simulink model "generic_uservehicle_truck"  (Simulink 10.3)
settings: Solver=ode45  StartTime=0.0  StopTime=inf  RelTol=1e-3  EnableMultiTasking=on
(part 4 of 4)

== system generic_uservehicle_truck/TruckMaker/Vehicle/IPG Vehicle/CarAndTrailer/Trailer/CreateBus Vhcl.Wheel.RL2 ==
  In1 : Inport
  Bus Creator3 : BusCreator  Inputs=14
  Demux3 : Demux  Outputs=14
      settings: DisplayOption=none
  Out1 : Outport  VectorParamsAs1DForOutWhenUnconnected=off
  wires:
  Demux3/14 -> Bus Creator3/14  "Vhcl Wheel RL2 Trq_WhlBearing"
  Demux3/13 -> Bus Creator3/13  "Vhcl Wheel RL2 Trq_T2W"
  Demux3/12 -> Bus Creator3/12  "Vhcl Wheel RL2 SideSlip"
  Demux3/11 -> Bus Creator3/11  "Vhcl Wheel RL2 LongSlip"
  Demux3/10 -> Bus Creator3/10  "Vhcl Wheel RL2 vBelt"
  Demux3/9 -> Bus Creator3/9  "Vhcl Wheel RL2 Fz"
  Demux3/8 -> Bus Creator3/8  "Vhcl Wheel RL2 Fy"
  Demux3/7 -> Bus Creator3/7  "Vhcl Wheel RL2 Fx"
  Demux3/6 -> Bus Creator3/6  "Vhcl Wheel RL2 r_zxy z"
  Demux3/5 -> Bus Creator3/5  "Vhcl Wheel RL2 r_zxy y"
  Demux3/4 -> Bus Creator3/4  "Vhcl Wheel RL2 r_zxy x"
  Demux3/3 -> Bus Creator3/3  "Vhcl Wheel RL2 t z"
  Demux3/2 -> Bus Creator3/2  "Vhcl Wheel RL2 t y"
  In1/1 -> Demux3/1
  Bus Creator3/1 -> Out1/1
  Demux3/1 -> Bus Creator3/1  "Vhcl Wheel RL2 t x"

== system generic_uservehicle_truck/TruckMaker/Vehicle/IPG Vehicle/CarAndTrailer/Trailer/CreateBus Vhcl.Wheel.RL3 ==
  In1 : Inport
  Bus Creator3 : BusCreator  Inputs=14
  Demux3 : Demux  Outputs=14
      settings: DisplayOption=none
  Out1 : Outport  VectorParamsAs1DForOutWhenUnconnected=off
  wires:
  Demux3/1 -> Bus Creator3/1  "Vhcl Wheel RL3 t x"
  Bus Creator3/1 -> Out1/1
  In1/1 -> Demux3/1
  Demux3/2 -> Bus Creator3/2  "Vhcl Wheel RL3 t y"
  Demux3/3 -> Bus Creator3/3  "Vhcl Wheel RL3 t z"
  Demux3/4 -> Bus Creator3/4  "Vhcl Wheel RL3 r_zxy x"
  Demux3/5 -> Bus Creator3/5  "Vhcl Wheel RL3 r_zxy y"
  Demux3/6 -> Bus Creator3/6  "Vhcl Wheel RL3 r_zxy z"
  Demux3/7 -> Bus Creator3/7  "Vhcl Wheel RL3 Fx"
  Demux3/8 -> Bus Creator3/8  "Vhcl Wheel RL3 Fy"
  Demux3/9 -> Bus Creator3/9  "Vhcl Wheel RL3 Fz"
  Demux3/10 -> Bus Creator3/10  "Vhcl Wheel RL3 vBelt"
  Demux3/11 -> Bus Creator3/11  "Vhcl Wheel RL3 LongSlip"
  Demux3/12 -> Bus Creator3/12  "Vhcl Wheel RL3 SideSlip"
  Demux3/13 -> Bus Creator3/13  "Vhcl Wheel RL3 Trq_T2W"
  Demux3/14 -> Bus Creator3/14  "Vhcl Wheel RL3 Trq_WhlBearing"

== system generic_uservehicle_truck/TruckMaker/Vehicle/IPG Vehicle/CarAndTrailer/Trailer/CreateBus Vhcl.Wheel.RL4 ==
  In1 : Inport
  Bus Creator3 : BusCreator  Inputs=14
  Demux3 : Demux  Outputs=14
      settings: DisplayOption=none
  Out1 : Outport  VectorParamsAs1DForOutWhenUnconnected=off
  wires:
  Demux3/14 -> Bus Creator3/14  "Vhcl Wheel RL4 Trq_WhlBearing"
  Demux3/13 -> Bus Creator3/13  "Vhcl Wheel RL4 Trq_T2W"
  Demux3/12 -> Bus Creator3/12  "Vhcl Wheel RL4 SideSlip"
  Demux3/11 -> Bus Creator3/11  "Vhcl Wheel RL4 LongSlip"
  Demux3/10 -> Bus Creator3/10  "Vhcl Wheel RL4 vBelt"
  Demux3/9 -> Bus Creator3/9  "Vhcl Wheel RL4 Fz"
  Demux3/8 -> Bus Creator3/8  "Vhcl Wheel RL4 Fy"
  Demux3/7 -> Bus Creator3/7  "Vhcl Wheel RL4 Fx"
  Demux3/6 -> Bus Creator3/6  "Vhcl Wheel RL4 r_zxy z"
  Demux3/5 -> Bus Creator3/5  "Vhcl Wheel RL4 r_zxy y"
  Demux3/4 -> Bus Creator3/4  "Vhcl Wheel RL4 r_zxy x"
  Demux3/3 -> Bus Creator3/3  "Vhcl Wheel RL4 t z"
  Demux3/2 -> Bus Creator3/2  "Vhcl Wheel RL4 t y"
  In1/1 -> Demux3/1
  Bus Creator3/1 -> Out1/1
  Demux3/1 -> Bus Creator3/1  "Vhcl Wheel RL4 t x"

== system generic_uservehicle_truck/TruckMaker/Vehicle/IPG Vehicle/CarAndTrailer/Trailer/CreateBus Vhcl.Wheel.RR ==
  In1 : Inport
  Bus Creator3 : BusCreator  Inputs=14
  Demux3 : Demux  Outputs=14
      settings: DisplayOption=none
  Out1 : Outport  VectorParamsAs1DForOutWhenUnconnected=off
  wires:
  Demux3/14 -> Bus Creator3/14  "Vhcl Wheel RR Trq_WhlBearing"
  Demux3/13 -> Bus Creator3/13  "Vhcl Wheel RR Trq_T2W"
  Demux3/12 -> Bus Creator3/12  "Vhcl Wheel RR SideSlip"
  Demux3/11 -> Bus Creator3/11  "Vhcl Wheel RR LongSlip"
  Demux3/10 -> Bus Creator3/10  "Vhcl Wheel RR vBelt"
  Demux3/9 -> Bus Creator3/9  "Vhcl Wheel RR Fz"
  Demux3/8 -> Bus Creator3/8  "Vhcl Wheel RR Fy"
  Demux3/7 -> Bus Creator3/7  "Vhcl Wheel RR Fx"
  Demux3/6 -> Bus Creator3/6  "Vhcl Wheel RR r_zxy z"
  Demux3/5 -> Bus Creator3/5  "Vhcl Wheel RR r_zxy y"
  Demux3/4 -> Bus Creator3/4  "Vhcl Wheel RR r_zxy x"
  Demux3/3 -> Bus Creator3/3  "Vhcl Wheel RR t z"
  Demux3/2 -> Bus Creator3/2  "Vhcl Wheel RR t y"
  In1/1 -> Demux3/1
  Bus Creator3/1 -> Out1/1
  Demux3/1 -> Bus Creator3/1  "Vhcl Wheel RR t x"

== system generic_uservehicle_truck/TruckMaker/Vehicle/IPG Vehicle/CarAndTrailer/Trailer/CreateBus Vhcl.Wheel.RR2 ==
  In1 : Inport
  Bus Creator3 : BusCreator  Inputs=14
  Demux3 : Demux  Outputs=14
      settings: DisplayOption=none
  Out1 : Outport  VectorParamsAs1DForOutWhenUnconnected=off
  wires:
  Demux3/14 -> Bus Creator3/14  "Vhcl Wheel RR2 Trq_WhlBearing"
  Demux3/13 -> Bus Creator3/13  "Vhcl Wheel RR2 Trq_T2W"
  Demux3/12 -> Bus Creator3/12  "Vhcl Wheel RR2 SideSlip"
  Demux3/11 -> Bus Creator3/11  "Vhcl Wheel RR2 LongSlip"
  Demux3/10 -> Bus Creator3/10  "Vhcl Wheel RR2 vBelt"
  Demux3/9 -> Bus Creator3/9  "Vhcl Wheel RR2 Fz"
  Demux3/8 -> Bus Creator3/8  "Vhcl Wheel RR2 Fy"
  Demux3/7 -> Bus Creator3/7  "Vhcl Wheel RR2 Fx"
  Demux3/6 -> Bus Creator3/6  "Vhcl Wheel RR2 r_zxy z"
  Demux3/5 -> Bus Creator3/5  "Vhcl Wheel RR2 r_zxy y"
  Demux3/4 -> Bus Creator3/4  "Vhcl Wheel RR2 r_zxy x"
  Demux3/3 -> Bus Creator3/3  "Vhcl Wheel RR2 t z"
  Demux3/2 -> Bus Creator3/2  "Vhcl Wheel RR2 t y"
  In1/1 -> Demux3/1
  Bus Creator3/1 -> Out1/1
  Demux3/1 -> Bus Creator3/1  "Vhcl Wheel RR2 t x"

== system generic_uservehicle_truck/TruckMaker/Vehicle/IPG Vehicle/CarAndTrailer/Trailer/CreateBus Vhcl.Wheel.RR3 ==
  In1 : Inport
  Bus Creator3 : BusCreator  Inputs=14
  Demux3 : Demux  Outputs=14
      settings: DisplayOption=none
  Out1 : Outport  VectorParamsAs1DForOutWhenUnconnected=off
  wires:
  Demux3/1 -> Bus Creator3/1  "Vhcl Wheel RR3 t x"
  Bus Creator3/1 -> Out1/1
  In1/1 -> Demux3/1
  Demux3/2 -> Bus Creator3/2  "Vhcl Wheel RR3 t y"
  Demux3/3 -> Bus Creator3/3  "Vhcl Wheel RR3 t z"
  Demux3/4 -> Bus Creator3/4  "Vhcl Wheel RR3 r_zxy x"
  Demux3/5 -> Bus Creator3/5  "Vhcl Wheel RR3 r_zxy y"
  Demux3/6 -> Bus Creator3/6  "Vhcl Wheel RR3 r_zxy z"
  Demux3/7 -> Bus Creator3/7  "Vhcl Wheel RR3 Fx"
  Demux3/8 -> Bus Creator3/8  "Vhcl Wheel RR3 Fy"
  Demux3/9 -> Bus Creator3/9  "Vhcl Wheel RR3 Fz"
  Demux3/10 -> Bus Creator3/10  "Vhcl Wheel RR3 vBelt"
  Demux3/11 -> Bus Creator3/11  "Vhcl Wheel RR3 LongSlip"
  Demux3/12 -> Bus Creator3/12  "Vhcl Wheel RR3 SideSlip"
  Demux3/13 -> Bus Creator3/13  "Vhcl Wheel RR3 Trq_T2W"
  Demux3/14 -> Bus Creator3/14  "Vhcl Wheel RR3 Trq_WhlBearing"

== system generic_uservehicle_truck/TruckMaker/Vehicle/IPG Vehicle/CarAndTrailer/Trailer/CreateBus Vhcl.Wheel.RR4 ==
  In1 : Inport
  Bus Creator3 : BusCreator  Inputs=14
  Demux3 : Demux  Outputs=14
      settings: DisplayOption=none
  Out1 : Outport  VectorParamsAs1DForOutWhenUnconnected=off
  wires:
  Demux3/14 -> Bus Creator3/14  "Vhcl Wheel RR4 Trq_WhlBearing"
  Demux3/13 -> Bus Creator3/13  "Vhcl Wheel RR4 Trq_T2W"
  Demux3/12 -> Bus Creator3/12  "Vhcl Wheel RR4 SideSlip"
  Demux3/11 -> Bus Creator3/11  "Vhcl Wheel RR4 LongSlip"
  Demux3/10 -> Bus Creator3/10  "Vhcl Wheel RR4 vBelt"
  Demux3/9 -> Bus Creator3/9  "Vhcl Wheel RR4 Fz"
  Demux3/8 -> Bus Creator3/8  "Vhcl Wheel RR4 Fy"
  Demux3/7 -> Bus Creator3/7  "Vhcl Wheel RR4 Fx"
  Demux3/6 -> Bus Creator3/6  "Vhcl Wheel RR4 r_zxy z"
  Demux3/5 -> Bus Creator3/5  "Vhcl Wheel RR4 r_zxy y"
  Demux3/4 -> Bus Creator3/4  "Vhcl Wheel RR4 r_zxy x"
  Demux3/3 -> Bus Creator3/3  "Vhcl Wheel RR4 t z"
  Demux3/2 -> Bus Creator3/2  "Vhcl Wheel RR4 t y"
  In1/1 -> Demux3/1
  Bus Creator3/1 -> Out1/1
  Demux3/1 -> Bus Creator3/1  "Vhcl Wheel RR4 t x"

== system generic_uservehicle_truck/TruckMaker/Vehicle/User Vehicle (CM4SL)/CarAndTrailer/CarAndTrailerUpd/CreateBus Brake.IF.In ==
  In : Inport
  BusCreator : BusCreator  Inputs=25
  Demux : Demux  Outputs=25
      settings: DisplayOption=none
  Out : Outport  VectorParamsAs1DForOutWhenUnconnected=off
  wires:
  Demux/25 -> BusCreator/25  "Brake IF Trq_Reg RR4"
  Demux/24 -> BusCreator/24  "Brake IF Trq_Reg RL4"
  Demux/23 -> BusCreator/23  "Brake IF Trq_Reg RR3"
  Demux/22 -> BusCreator/22  "Brake IF Trq_Reg RL3"
  Demux/21 -> BusCreator/21  "Brake IF Trq_Reg FR2"
  Demux/20 -> BusCreator/20  "Brake IF Trq_Reg FL2"
  Demux/19 -> BusCreator/19  "Brake IF Trq_Reg RR2"
  Demux/18 -> BusCreator/18  "Brake IF Trq_Reg RL2"
  Demux/17 -> BusCreator/17  "Brake IF Trq_Reg RR"
  Demux/16 -> BusCreator/16  "Brake IF Trq_Reg RL"
  Demux/15 -> BusCreator/15  "Brake IF Trq_Reg FR"
  Demux/14 -> BusCreator/14  "Brake IF Trq_Reg FL"
  Demux/13 -> BusCreator/13  "Brake IF Trq_Reg_max RR4"
  Demux/12 -> BusCreator/12  "Brake IF Trq_Reg_max RL4"
  Demux/11 -> BusCreator/11  "Brake IF Trq_Reg_max RR3"
  Demux/10 -> BusCreator/10  "Brake IF Trq_Reg_max RL3"
  Demux/9 -> BusCreator/9  "Brake IF Trq_Reg_max FR2"
  Demux/8 -> BusCreator/8  "Brake IF Trq_Reg_max FL2"
  Demux/7 -> BusCreator/7  "Brake IF Trq_Reg_max RR2"
  Demux/6 -> BusCreator/6  "Brake IF Trq_Reg_max RL2"
  Demux/5 -> BusCreator/5  "Brake IF Trq_Reg_max RR"
  Demux/4 -> BusCreator/4  "Brake IF Trq_Reg_max RL"
  Demux/3 -> BusCreator/3  "Brake IF Trq_Reg_max FR"
  Demux/2 -> BusCreator/2  "Brake IF Trq_Reg_max FL"
  Demux/1 -> BusCreator/1  "Brake IF T_env"
  BusCreator/1 -> Out/1
  In/1 -> Demux/1

== system generic_uservehicle_truck/TruckMaker/Vehicle/User Vehicle (ModelMgr)/CarAndTrailer/CarAndTrailerUpd/CreateBus Brake.IF.In ==
  In : Inport
  BusCreator : BusCreator  Inputs=25
  Demux : Demux  Outputs=25
      settings: DisplayOption=none
  Out : Outport  VectorParamsAs1DForOutWhenUnconnected=off
  wires:
  Demux/25 -> BusCreator/25  "Brake IF Trq_Reg RR4"
  Demux/24 -> BusCreator/24  "Brake IF Trq_Reg RL4"
  Demux/23 -> BusCreator/23  "Brake IF Trq_Reg RR3"
  Demux/22 -> BusCreator/22  "Brake IF Trq_Reg RL3"
  Demux/21 -> BusCreator/21  "Brake IF Trq_Reg FR2"
  Demux/20 -> BusCreator/20  "Brake IF Trq_Reg FL2"
  Demux/19 -> BusCreator/19  "Brake IF Trq_Reg RR2"
  Demux/18 -> BusCreator/18  "Brake IF Trq_Reg RL2"
  Demux/17 -> BusCreator/17  "Brake IF Trq_Reg RR"
  Demux/16 -> BusCreator/16  "Brake IF Trq_Reg RL"
  Demux/15 -> BusCreator/15  "Brake IF Trq_Reg FR"
  Demux/14 -> BusCreator/14  "Brake IF Trq_Reg FL"
  Demux/13 -> BusCreator/13  "Brake IF Trq_Reg_max RR4"
  Demux/12 -> BusCreator/12  "Brake IF Trq_Reg_max RL4"
  Demux/11 -> BusCreator/11  "Brake IF Trq_Reg_max RR3"
  Demux/10 -> BusCreator/10  "Brake IF Trq_Reg_max RL3"
  Demux/9 -> BusCreator/9  "Brake IF Trq_Reg_max FR2"
  Demux/8 -> BusCreator/8  "Brake IF Trq_Reg_max FL2"
  Demux/7 -> BusCreator/7  "Brake IF Trq_Reg_max RR2"
  Demux/6 -> BusCreator/6  "Brake IF Trq_Reg_max RL2"
  Demux/5 -> BusCreator/5  "Brake IF Trq_Reg_max RR"
  Demux/4 -> BusCreator/4  "Brake IF Trq_Reg_max RL"
  Demux/3 -> BusCreator/3  "Brake IF Trq_Reg_max FR"
  Demux/2 -> BusCreator/2  "Brake IF Trq_Reg_max FL"
  Demux/1 -> BusCreator/1  "Brake IF T_env"
  BusCreator/1 -> Out/1
  In/1 -> Demux/1
